simulink model "TriggerEdge2"  (R2020a)
settings: Solver=FixedStepAuto  StartTime=0.0  StopTime=10.0  FixedStep=0.1  MaxStep=1  RelTol=1e-3
settings Model: Creator=86188  LastModifiedBy=bzhan
settings DataIOCC: ReturnWorkspaceOutputs=off
settings DebuggingCC: ArithmeticOperatorsInVariantConditions=warning
settings SFSimCC: SimUseLocalCustomCode=off  CustomCodeUndefinedFunction=UseInterfaceOnly
settings RTWCC: RTWUseLocalCustomCode=off

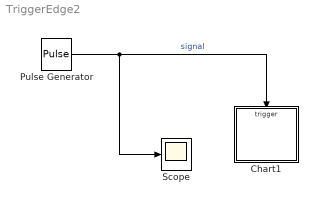
== system TriggerEdge2 ==
  Chart1 : Stateflow chart  TreatAsAtomicUnit=on
  Pulse Generator : DiscretePulseGenerator  PulseType=Time based  Period=1  PulseWidth=50
  Scope : Scope
  wires:
  Pulse Generator/1 -> Chart1/Trigger, Scope/1  "signal"

== stateflow chart TriggerEdge2/Chart1 ==
  state AA
    en:f("en_AA");
    du:f("du_AA");
  (default) -> AA : {y = y + 1;}
  data: s function_input; y local =0
  events: out_cmd input FALLING_EDGE_EVENT
  function f(s):
    | function f(s)
    |   fprintf(s+"\n");
